simulink model "demo_zynq"  (R2019b)
settings: Solver=FixedStepAuto  StartTime=0.0  StopTime=0.02  RelTol=1e-3  EnableMultiTasking=on
InitFcn:
  | Ts_FPGA = 1/25e6;   % FPGA sampling time (clock)
  | Ts_ADC_comm = 1/2.5e6;   % ADC communication period
  | Ts_ADC_sample = 70e-6;   % ADC sampling time
  | 
  | Ts_ARM = 210e-6;   % ARM execution period
  | 
  | DeadTime = 1e-6;   % deadtime for output signals
  | 
  | FIFO_length = 1000;   % number of fifo samples
  | 
  | Ts_SRO = 1/8e6; % communication time for the shift register outputs
model workspace (MAT data in the model file):
  mwTaskManagerKernelLatency = 1e-06
undefined symbols (not defined in the file): pos_bit
libraries: simulink x43, hdlsllib x24
(part 2 of 2)

== matlab function demo_zynq/FPGA/balanced delays/FIFO_DataAcquisition/Debug_FIFO1/FIFO_Controller ==
  data: enableFIFO input; pushFIFO input; fifo_push output; fifo_pop output; enableRead input; popFIFO input; fifo_full input; fifo_empty input; ignore output
function [fifo_push, fifo_pop, ignore] = fcn(enableFIFO, pushFIFO, enableRead, popFIFO, fifo_full, fifo_empty)
%#codegen

fifo_push = false;
fifo_pop = false;
ignore = true;

if enableFIFO
    
    if enableRead     
        % start poping
        ignore = false;
        if popFIFO && ~fifo_empty
            fifo_pop = true;
        end
        if fifo_empty
            ignore = true;
        end
    else
        % start loging
        ignore = true;
        if pushFIFO
            fifo_push = true;
            if fifo_full
                fifo_pop = true;                
            end
        end
    end
    
end

== matlab function demo_zynq/FPGA/balanced delays/FIFO_DataAcquisition/Debug_FIFO/FIFO_Controller ==
  data: enableFIFO input; pushFIFO input; fifo_push output; fifo_pop output; enableRead input; popFIFO input; fifo_full input; fifo_empty input; ignore output
function [fifo_push, fifo_pop, ignore] = fcn(enableFIFO, pushFIFO, enableRead, popFIFO, fifo_full, fifo_empty)
%#codegen

fifo_push = false;
fifo_pop = false;
ignore = true;

if enableFIFO
    
    if enableRead     
        % start poping
        ignore = false;
        if popFIFO && ~fifo_empty
            fifo_pop = true;
        end
        if fifo_empty
            ignore = true;
        end
    else
        % start loging
        ignore = true;
        if pushFIFO
            fifo_push = true;
            if fifo_full
                fifo_pop = true;                
            end
        end
    end
    
end

== matlab function demo_zynq/FPGA/balanced delays/FIFO_DataAcquisition/Debug_FIFO2/FIFO_Controller ==
  data: enableFIFO input; pushFIFO input; fifo_push output; fifo_pop output; enableRead input; popFIFO input; fifo_full input; fifo_empty input; ignore output
function [fifo_push, fifo_pop, ignore] = fcn(enableFIFO, pushFIFO, enableRead, popFIFO, fifo_full, fifo_empty)
%#codegen

fifo_push = false;
fifo_pop = false;
ignore = true;

if enableFIFO
    
    if enableRead     
        % start poping
        ignore = false;
        if popFIFO && ~fifo_empty
            fifo_pop = true;
        end
        if fifo_empty
            ignore = true;
        end
    else
        % start loging
        ignore = true;
        if pushFIFO
            fifo_push = true;
            if fifo_full
                fifo_pop = true;                
            end
        end
    end
    
end

== matlab function demo_zynq/FPGA/balanced delays/FIFO_DataAcquisition/Debug_FIFO3/FIFO_Controller ==
  data: enableFIFO input; pushFIFO input; fifo_push output; fifo_pop output; enableRead input; popFIFO input; fifo_full input; fifo_empty input; ignore output
function [fifo_push, fifo_pop, ignore] = fcn(enableFIFO, pushFIFO, enableRead, popFIFO, fifo_full, fifo_empty)
%#codegen

fifo_push = false;
fifo_pop = false;
ignore = true;

if enableFIFO
    
    if enableRead     
        % start poping
        ignore = false;
        if popFIFO && ~fifo_empty
            fifo_pop = true;
        end
        if fifo_empty
            ignore = true;
        end
    else
        % start loging
        ignore = true;
        if pushFIFO
            fifo_push = true;
            if fifo_full
                fifo_pop = true;                
            end
        end
    end
    
end
